simulink model "Input_Event_2018a"  (R2018a)
settings: Solver=VariableStepAuto  StartTime=0.0  StopTime=10.0  RelTol=1e-3
settings Model: Creator=apple  LastModifiedBy=BEAR
settings DataIOCC: ReturnWorkspaceOutputs=on
settings SFSimCC: SimUseLocalCustomCode=on
settings RTWCC: RTWUseLocalCustomCode=on

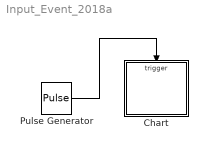
== system Input_Event_2018a ==
  Chart : Stateflow chart  TreatAsAtomicUnit=on
  Pulse Generator : DiscretePulseGenerator  PulseType=Time based  Period=10  PulseWidth=50
  wires:
  Pulse Generator/1 -> Chart/Trigger

== stateflow chart Input_Event_2018a/Chart ==
  state On2
    en:fprintf("Entry_On");
    du:fprintf("During_On");
    ex:fprintf("Exit_On");
  state On
    en:fprintf("Entry_On");
    du:fprintf("During_On");
    ex:fprintf("Exit_On");
  state Off
    en:fprintf("Entry_Off");
    du:fprintf("During_Off");
    ex:fprintf("Exit_Off");
  (default) -> On
  On -> On2 [order 2] : E
  On -> Off [order 1] : E_one/{send(E);}
  events: E_one input EITHER_EDGE_EVENT; E local FUNCTION_CALL_EVENT
